simulink model "IDEALMOTORVAL"  (R2023a)
settings: Solver=VariableStepAuto  StartTime=0.0  StopTime=10  RelTol=1e-3
values from neighbouring files (symbols this model uses):
  A = [0,-k/2;1/(2*m),-b/(4*m)]    [IDEALMOTOR.m]    (also in Pittman_step.m)
  B = [k*r/2,0; b*r/(4*m),1/m]    [IDEALMOTOR.m]    (also in Pittman_step.m)
  C = eye(2)    [IDEALMOTOR.m]    (also in Pittman_step.m)
  D = [0,0;0,0]    [IDEALMOTOR.m]    (also in Pittman_step.m)
  g = 9.81    [IDEALMOTOR.m]    (also in Pittman_step.m)
  m = 1    [IDEALMOTOR.m]    (also in Pittman_step.m)
  N = 5.9    [IDEALMOTOR.m]    (also in Pittman_step.m)
  tau = 0.05    [IDEALMOTOR.m]    (also in Pittman_step.m)
libraries: cstblocks x1
settings Model: Creator=Administrator  LastModifiedBy=Administrator

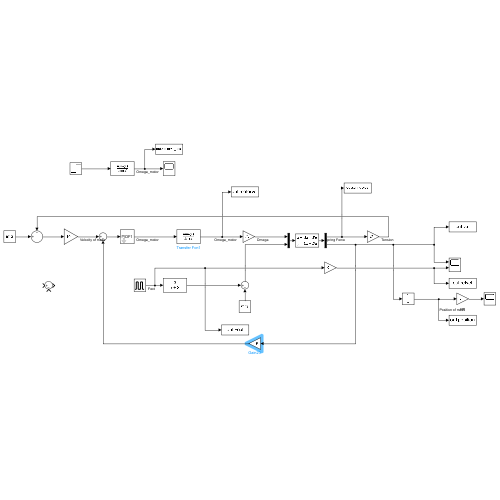
[thumbnail: Simulink's stored preview of the top-level diagram]
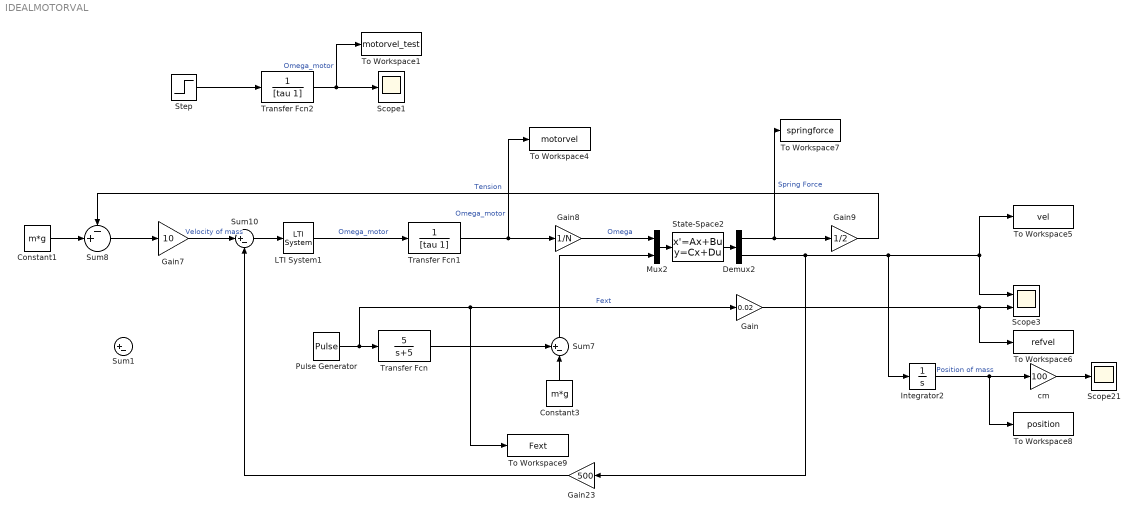
== system IDEALMOTORVAL ==
  Constant1 : Constant  Value=m*g
  Constant3 : Constant  Value=m*g
  Demux2 : Demux  Outputs=2
  Gain : Gain  Gain=0.02
  Gain23 : Gain  Gain=500
  Gain7 : Gain  Gain=10
  Gain8 : Gain  Gain=1/N
  Gain9 : Gain  Gain=1/2
  Integrator2 : Integrator
  LTI System1 : cstblocks/LTI System  sys=PIDF1  IC=[]
  Mux2 : Mux  Inputs=2
  Pulse Generator : DiscretePulseGenerator  PulseType=Time based  Amplitude=7.5  Period=5  PulseWidth=50
  Scope1 : Scope
  Scope21 : Scope
  Scope3 : Scope  NumInputPorts=2
  State-Space2 : StateSpace  A=A  B=B  C=C  D=D  InitialCondition=[2*m*g 0]
  Step : Step  Time=0  After=104  SampleTime=0
  Sum1 : Sum  Inputs=|+-
  Sum10 : Sum  Inputs=|+-
  Sum7 : Sum  Inputs=+-|
  Sum8 : Sum  Inputs=-+|
  To Workspace1 : ToWorkspace  VariableName=motorvel_test  SaveFormat=Timeseries  SampleTime=-1
  To Workspace4 : ToWorkspace  VariableName=motorvel  SaveFormat=Timeseries  SampleTime=-1
  To Workspace5 : ToWorkspace  VariableName=vel  SaveFormat=Timeseries  SampleTime=-1
  To Workspace6 : ToWorkspace  VariableName=refvel  SaveFormat=Timeseries  SampleTime=-1
  To Workspace7 : ToWorkspace  VariableName=springforce  SaveFormat=Timeseries  SampleTime=-1
  To Workspace8 : ToWorkspace  VariableName=position  SaveFormat=Timeseries  SampleTime=-1
  To Workspace9 : ToWorkspace  VariableName=Fext  SaveFormat=Timeseries  SampleTime=-1
  Transfer Fcn : TransferFcn  Numerator=[5]  Denominator=[1 5]
  Transfer Fcn1 : TransferFcn  Denominator=[tau 1]
  Transfer Fcn2 : TransferFcn  Denominator=[tau 1]
  cm : Gain  Gain=100
  wires:
  Transfer Fcn/1 -> Sum7/1
  LTI System1/1 -> Transfer Fcn1/1  "Omega_motor"
  Sum8/1 -> Gain7/1
  Sum7/1 -> Mux2/2
  Pulse Generator/1 -> To Workspace9/1, Gain/1, Transfer Fcn/1  "Fext"
  Integrator2/1 -> To Workspace8/1, cm/1  "Position of mass"
  Sum10/1 -> LTI System1/1
  Demux2/1 -> Gain9/1, To Workspace7/1  "Spring Force"
  Mux2/1 -> State-Space2/1
  Gain7/1 -> Sum10/1  "Velocity of mass"
  Gain9/1 -> Sum8/1  "Tension"
  Constant3/1 -> Sum7/2
  Gain23/1 -> Sum10/2
  Constant1/1 -> Sum8/2
  Gain/1 -> To Workspace6/1, Scope3/2
  Transfer Fcn1/1 -> Gain8/1, To Workspace4/1  "Omega_motor"
  Gain8/1 -> Mux2/1  "Omega"
  State-Space2/1 -> Demux2/1
  Demux2/2 -> To Workspace5/1, Scope3/1, Integrator2/1, Gain23/1
  cm/1 -> Scope21/1
  Step/1 -> Transfer Fcn2/1
  Transfer Fcn2/1 -> To Workspace1/1, Scope1/1  "Omega_motor"
